simulink model "bo1808_svpwm_sim"  (R2024b)
settings: Solver=ode23tb  StartTime=0.0  StopTime=t_stop_svpwm  MaxStep=Ts_sim_svpwm  RelTol=1e-3
model workspace (MAT data in the model file):
  Ts_pwm_svpwm = 5e-05
  Ts_sim_svpwm = 1e-06
  Uref_svpwm = 4.83590678003
  Vdc = 11.4
  Vref_max_svpwm = 6.58179306876
  f_ref_svpwm = 519.333333333
  fft_cycles_svpwm = 20
  fs_pwm = 20000
  id_ref_svpwm = 0
  iq_ref_svpwm = 0.1875
  m_svpwm = 0.734740021375
  omega_ref_svpwm = 3263.06756953
  t_stop_svpwm = 0.0385109114249
  ud_ref_svpwm = -0.226375312636
  uq_ref_svpwm = 4.8306054075
libraries: simulink x1
settings Model: Creator=26683  LastModifiedBy=26683

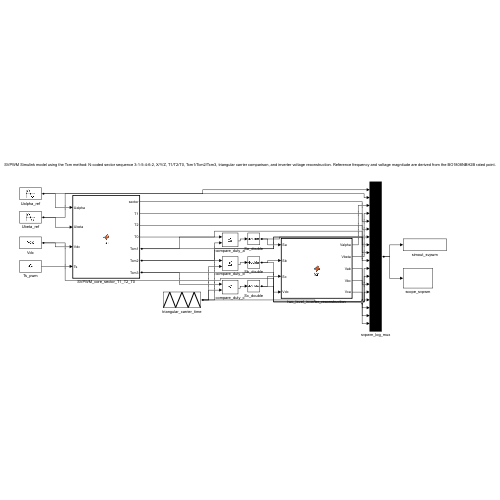
[thumbnail: Simulink's stored preview of the top-level diagram]
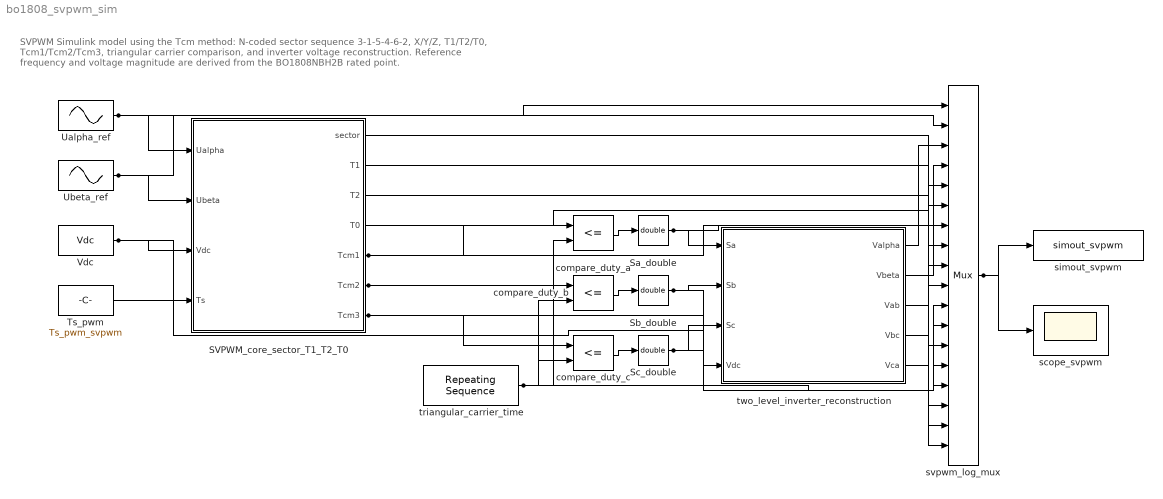
== system bo1808_svpwm_sim ==
  note: SVPWM Simulink model using the Tcm method: N-coded sector sequence 3-1-5-4-6-2, X/Y/Z, T1/T2/T0, Tcm1/Tcm2/Tcm3, triangular carrier comparison, and inverter voltage reconstruction. Reference frequency and voltage magnitude are derived from the BO1808NBH2B rated point.
  SVPWM_core_sector_T1_T2_T0 : MATLAB Function  TreatAsAtomicUnit=on
  Sa_double : DataTypeConversion  OutDataTypeStr=double  SaturateOnIntegerOverflow=off  RndMeth=Floor
  Sb_double : DataTypeConversion  OutDataTypeStr=double  SaturateOnIntegerOverflow=off  RndMeth=Floor
  Sc_double : DataTypeConversion  OutDataTypeStr=double  SaturateOnIntegerOverflow=off  RndMeth=Floor
  Ts_pwm : Constant  Value=Ts_pwm_svpwm
  Ualpha_ref : Sin  Amplitude=Uref_svpwm  Frequency=2*pi*f_ref_svpwm  Phase=pi/2  SampleTime=0
  Ubeta_ref : Sin  Amplitude=Uref_svpwm  Frequency=2*pi*f_ref_svpwm  SampleTime=0
  Vdc : Constant  Value=Vdc
  compare_duty_a : RelationalOperator  Operator=<=  OutDataTypeStr=boolean  RndMeth=Simplest  InputSameDT=off
  compare_duty_b : RelationalOperator  Operator=<=  OutDataTypeStr=boolean  RndMeth=Simplest  InputSameDT=off
  compare_duty_c : RelationalOperator  Operator=<=  OutDataTypeStr=boolean  RndMeth=Simplest  InputSameDT=off
  scope_svpwm : Scope
  simout_svpwm : ToWorkspace  VariableName=simout_svpwm  SaveFormat=Structure With Time  SampleTime=-1
  svpwm_log_mux : Mux  Inputs=18
  triangular_carrier_time : simulink/Sources/Repeating Sequence  rep_seq_t=[0 Ts_pwm_svpwm/2 Ts_pwm_svpwm]  rep_seq_y=[0 Ts_pwm_svpwm/2 0]
  two_level_inverter_reconstruction : MATLAB Function  TreatAsAtomicUnit=on
  wires:
  Ualpha_ref/1 -> SVPWM_core_sector_T1_T2_T0/1(Ualpha), svpwm_log_mux/1
  Ubeta_ref/1 -> SVPWM_core_sector_T1_T2_T0/2(Ubeta), svpwm_log_mux/2
  Vdc/1 -> SVPWM_core_sector_T1_T2_T0/3(Vdc), two_level_inverter_reconstruction/4(Vdc)
  Ts_pwm/1 -> SVPWM_core_sector_T1_T2_T0/4(Ts)
  SVPWM_core_sector_T1_T2_T0/5(Tcm1) -> compare_duty_a/1, svpwm_log_mux/9
  SVPWM_core_sector_T1_T2_T0/6(Tcm2) -> compare_duty_b/1, svpwm_log_mux/10
  SVPWM_core_sector_T1_T2_T0/7(Tcm3) -> compare_duty_c/1, svpwm_log_mux/11
  triangular_carrier_time/1 -> compare_duty_a/2, compare_duty_b/2, compare_duty_c/2, svpwm_log_mux/12
  compare_duty_a/1 -> Sa_double/1
  compare_duty_b/1 -> Sb_double/1
  compare_duty_c/1 -> Sc_double/1
  Sa_double/1 -> two_level_inverter_reconstruction/1(Sa), svpwm_log_mux/13
  Sb_double/1 -> two_level_inverter_reconstruction/2(Sb), svpwm_log_mux/14
  Sc_double/1 -> two_level_inverter_reconstruction/3(Sc), svpwm_log_mux/15
  two_level_inverter_reconstruction/1(Valpha) -> svpwm_log_mux/3
  two_level_inverter_reconstruction/2(Vbeta) -> svpwm_log_mux/4
  SVPWM_core_sector_T1_T2_T0/1(sector) -> svpwm_log_mux/5
  SVPWM_core_sector_T1_T2_T0/2(T1) -> svpwm_log_mux/6
  SVPWM_core_sector_T1_T2_T0/3(T2) -> svpwm_log_mux/7
  SVPWM_core_sector_T1_T2_T0/4(T0) -> svpwm_log_mux/8
  two_level_inverter_reconstruction/3(Vab) -> svpwm_log_mux/16
  two_level_inverter_reconstruction/4(Vbc) -> svpwm_log_mux/17
  two_level_inverter_reconstruction/5(Vca) -> svpwm_log_mux/18
  svpwm_log_mux/1 -> simout_svpwm/1, scope_svpwm/1

== matlab function bo1808_svpwm_sim/two_level_inverter_reconstruction ==
  data: Sa input; Valpha output; Sb input; Sc input; Vdc input; Vbeta output; Vab output; Vbc output; Vca output
function [Valpha,Vbeta,Vab,Vbc,Vca] = fcn(Sa,Sb,Sc,Vdc)
%#codegen
sa = double(Sa);
sb = double(Sb);
sc = double(Sc);
Va0 = (sa - 0.5)*Vdc;
Vb0 = (sb - 0.5)*Vdc;
Vc0 = (sc - 0.5)*Vdc;
Vab = Va0 - Vb0;
Vbc = Vb0 - Vc0;
Vca = Vc0 - Va0;
Valpha = (2/3)*(Va0 - 0.5*Vb0 - 0.5*Vc0);
Vbeta = (2/3)*(sqrt(3)/2)*(Vb0 - Vc0);
end

== matlab function bo1808_svpwm_sim/SVPWM_core_sector_T1_T2_T0 ==
  data: Ualpha input; sector output; Ubeta input; Vdc input; Ts input; T1 output; T2 output; T0 output; Tcm1 output; Tcm2 output; Tcm3 output
function [sector,T1,T2,T0,Tcm1,Tcm2,Tcm3] = fcn(Ualpha,Ubeta,Vdc,Ts)
%#codegen
Vref1 = Ubeta;
Vref2 = (sqrt(3)*Ualpha - Ubeta)/2;
Vref3 = (-sqrt(3)*Ualpha - Ubeta)/2;
A = 0;
B = 0;
C = 0;
if Vref1 >= 0
    A = 1;
end
if Vref2 >= 0
    B = 1;
end
if Vref3 >= 0
    C = 1;
end
sector = 4*C + 2*B + A;
if sector < 1
    sector = 1;
end
X = sqrt(3)*Ubeta*Ts/Vdc;
Y = Ts/Vdc*(1.5*Ualpha + sqrt(3)/2*Ubeta);
Z = Ts/Vdc*(-1.5*Ualpha + sqrt(3)/2*Ubeta);
if sector == 1
    T1 = Z;
    T2 = Y;
elseif sector == 2
    T1 = Y;
    T2 = -X;
elseif sector == 3
    T1 = -Z;
    T2 = X;
elseif sector == 4
    T1 = -X;
    T2 = Z;
elseif sector == 5
    T1 = X;
    T2 = -Y;
else
    T1 = -Y;
    T2 = -Z;
end
if T1 < 0
    T1 = 0;
end
if T2 < 0
    T2 = 0;
end
if T1 + T2 > Ts
    scale = Ts/(T1 + T2);
    T1 = T1*scale;
    T2 = T2*scale;
end
T0 = Ts - T1 - T2;
ta = T0/4;
tb = ta + T1/2;
tc = tb + T2/2;
if sector == 1
    Tcm1 = tb;
    Tcm2 = ta;
    Tcm3 = tc;
elseif sector == 2
    Tcm1 = ta;
    Tcm2 = tc;
    Tcm3 = tb;
elseif sector == 3
    Tcm1 = ta;
    Tcm2 = tb;
    Tcm3 = tc;
elseif sector == 4
    Tcm1 = tc;
    Tcm2 = tb;
    Tcm3 = ta;
elseif sector == 5
    Tcm1 = tc;
    Tcm2 = ta;
    Tcm3 = tb;
else
    Tcm1 = tb;
    Tcm2 = tc;
    Tcm3 = ta;
end
Tcm1 = min(max(Tcm1,0),Ts/2);
Tcm2 = min(max(Tcm2,0),Ts/2);
Tcm3 = min(max(Tcm3,0),Ts/2);
end
